simulink model "FiltroV3"  (R2024b)
settings: Solver=VariableStepAuto  StartTime=0.0  StopTime=inf  RelTol=1e-3
libraries: dspfdesign x5, dspsnks4 x1, dspvision x1
settings Model: Creator=fredy  LastModifiedBy=fredy

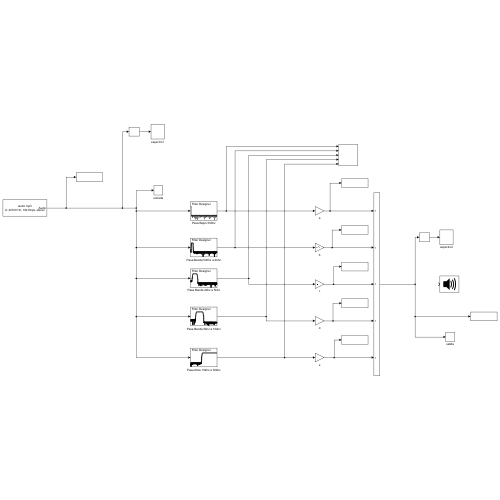
[thumbnail: Simulink's stored preview of the top-level diagram]
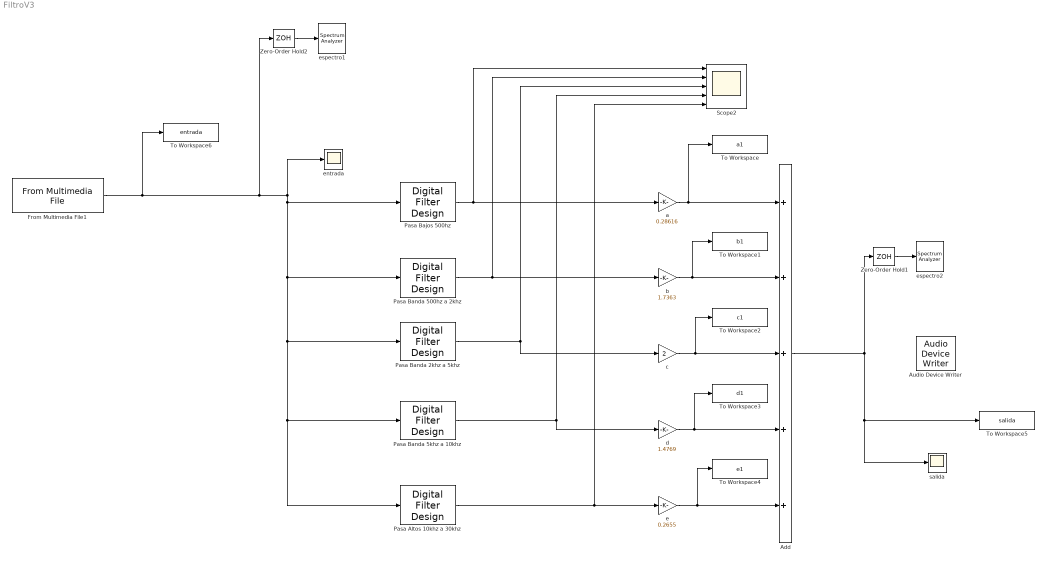
== system FiltroV3 ==
  Add : Sum  Inputs=+++++
  Audio Device Writer : dspsnks4/Audio Device Writer  Driver=DirectSound  Device=Default  InheritSampleRate=on  SampleRate=44100  BitDepth=16-bit integer  BufferSize=4096  NumBuffers=10  DefaultOutputChannelMapping=on  OutputChannelMapping=1:2  OutputNumUnderrunSamples=off  DriverIdx=1  DeviceWarnFlag=''
  From Multimedia File1 : dspvision/From Multimedia File  inputFilename=D:\Datos Fredy\Programacion\Matlab\Filtros\audio.mp3  readRange=[1 Inf]  loop=on  numPlays=inf  outputStreams=Audio only  videoDataType=single  audioDataType=single  inheritSampleTime=on  userDefinedSampleTime=1/30  noAudioOutput=off  isIntensityVideo=off  fourcc=RGB  colorVideoFormat=Separate color signals  outputEOF=off  dataOrg=Column-major  audioFrameSize=1  computeAudioFrameSize=off  outSamplingMode=Sample based
      settings: LibrarySourceBlock=audiosources/From Multimedia File
  Pasa Altos 10khz a 30khz : dspfdesign/Digital Filter Design  mwdsp_browser_bugfix_var=off
  Pasa Bajos 500hz : dspfdesign/Digital Filter Design  mwdsp_browser_bugfix_var=off
  Pasa Banda 2khz a 5khz : dspfdesign/Digital Filter Design  mwdsp_browser_bugfix_var=off
  Pasa Banda 500hz a 2khz : dspfdesign/Digital Filter Design  mwdsp_browser_bugfix_var=off
  Pasa Banda 5khz a 10khz : dspfdesign/Digital Filter Design  mwdsp_browser_bugfix_var=off
  Scope2 : Scope  NumInputPorts=5
  To Workspace : ToWorkspace  VariableName=a1  SaveFormat=Timeseries  SampleTime=-1
  To Workspace1 : ToWorkspace  VariableName=b1  SaveFormat=Timeseries  SampleTime=-1
  To Workspace2 : ToWorkspace  VariableName=c1  SaveFormat=Timeseries  SampleTime=-1
  To Workspace3 : ToWorkspace  VariableName=d1  SaveFormat=Timeseries  SampleTime=-1
  To Workspace4 : ToWorkspace  VariableName=e1  SaveFormat=Timeseries  SampleTime=-1
  To Workspace5 : ToWorkspace  VariableName=salida  SaveFormat=Timeseries  SampleTime=-1
  To Workspace6 : ToWorkspace  VariableName=entrada  SaveFormat=Timeseries  SampleTime=-1
  Zero-Order Hold1 : ZeroOrderHold  SampleTime=0.0001
  Zero-Order Hold2 : ZeroOrderHold  SampleTime=0.0001
  a : Gain  Gain=0.28616
  b : Gain  Gain=1.7363
  c : Gain  Gain=2
  d : Gain  Gain=1.4769
  e : Gain  Gain=0.2655
  entrada : Scope
  espectro1 : SpectrumAnalyzer  WindowPosition=[1044.000000,429.000000,1132.000000,626.000000,]  Visible=on  ScopeFrameLocation=window  SampleRate=44.1e3  PlotAsTwoSidedSpectrum=off  FrequencyScale=Log  WindowInvariantSamplesPerUpdate=on  FrequencySpan=Start and stop frequencies  StartFrequency=20  YLimits=[-48.94684797,13.76730878]  SelectedToolstripTab=spectrumAnalyzerToolstrip.estimationTab
  espectro2 : SpectrumAnalyzer  WindowPosition=[1027.000000,378.000000,1132.000000,626.000000,]  Visible=on  ScopeFrameLocation=window  SampleRate=44.1e3  PlotAsTwoSidedSpectrum=off  FrequencyScale=Log  WindowInvariantSamplesPerUpdate=on  FrequencySpan=Start and stop frequencies  StartFrequency=20  YLimits=[-47.91227719,14.00488228]
  salida : Scope
  wires:
  From Multimedia File1/1 -> To Workspace6/1, Zero-Order Hold2/1, Pasa Banda 500hz a 2khz/1, Pasa Banda 2khz a 5khz/1, Pasa Altos 10khz a 30khz/1, Pasa Banda 5khz a 10khz/1, Pasa Bajos 500hz/1, entrada/1
  Zero-Order Hold2/1 -> espectro1/1
  Pasa Banda 2khz a 5khz/1 -> c/1, Scope2/3
  Pasa Banda 5khz a 10khz/1 -> d/1, Scope2/4
  Pasa Altos 10khz a 30khz/1 -> e/1, Scope2/5
  Pasa Banda 500hz a 2khz/1 -> b/1, Scope2/2
  Pasa Bajos 500hz/1 -> a/1, Scope2/1
  Add/1 -> To Workspace5/1, salida/1, Zero-Order Hold1/1
  Zero-Order Hold1/1 -> espectro2/1
  b/1 -> To Workspace1/1, Add/2
  c/1 -> To Workspace2/1, Add/3
  d/1 -> To Workspace3/1, Add/4
  e/1 -> To Workspace4/1, Add/5
  a/1 -> To Workspace/1, Add/1
